simulink model "controller"  (R2019b)
settings: Solver=FixedStepAuto  StartTime=0.0  StopTime=10.0  RelTol=1e-3
undefined symbols (not defined in the file): Kd_mat, Kp_mat
settings Model: Creator=LBRY-SVC-Patron  LastModifiedBy=logan
settings DataIOCC: ReturnWorkspaceOutputs=off
settings OptimizationCC: DefaultParameterBehavior=Inlined  UseDivisionForNetSlopeComputation=on  GainParamInheritBuiltInType=on  UseFloatMulNetSlope=on  InlineInvariantSignals=on  PassReuseOutputArgsAs=Individual arguments  ZeroExternalMemoryAtStartup=off  ZeroInternalMemoryAtStartup=off  NoFixptDivByZeroProtection=on  EfficientFloat2IntCast=on  LifeSpan=1  EfficientTunableParamExpr=on
settings DebuggingCC: ParameterTunabilityLossMsg=error  ArithmeticOperatorsInVariantConditions=warning
settings HardwareCC: ProdLongLongMode=on
settings SFSimCC: SimUseLocalCustomCode=off  MATLABDynamicMemAlloc=off  CustomCodeUndefinedFunction=UseInterfaceOnly
settings RTWCC: SystemTargetFile=ert.tlc  TemplateMakefile=ert_default_tmf  GenerateReport=on  RTWUseLocalCustomCode=off  IncludeHyperlinkInReport=on  LaunchReport=on  TargetLang=C++  GenerateTraceInfo=on  GenerateTraceReport=on  GenerateTraceReportSl=on  GenerateTraceReportSf=on  GenerateTraceReportEml=on
settings CodeAppCC: ForceParamTrailComments=on  IgnoreCustomStorageClasses=off  OperatorAnnotations=on  SimulinkDataObjDesc=on  SFDataObjDesc=on  InsertBlockDesc=on
settings ERTTargetCC: TargetLangStandard=C++03 (ISO)  GenerateSampleERTMain=on  IncludeMdlTerminateFcn=off  CombineSignalStateStructs=on  MultiInstanceERTCode=on  CodeInterfacePackaging=C++ class  SupportComplex=off  SupportContinuousTime=on  InlinedParameterPlacement=NonHierarchical  RootIOFormat=Structure reference  ERTCustomFileTemplate=example_file_process.tlc  ERTFilePackagingFormat=CompactWithDataFile

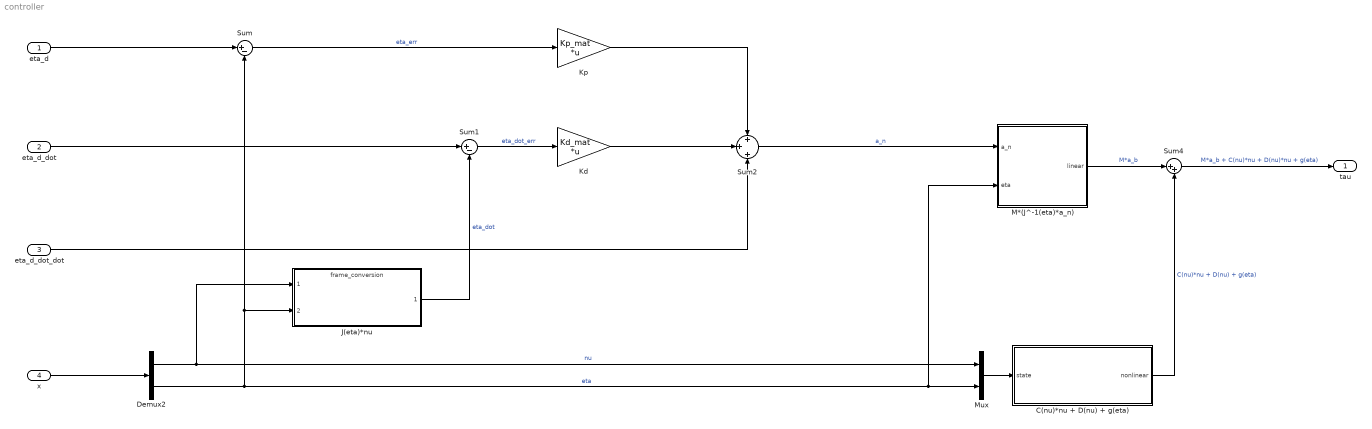
== system controller ==
  eta_d : Inport  PortDimensions=6
  eta_d_dot : Inport  Port=2  PortDimensions=6
  eta_d_dot_dot : Inport  Port=3  PortDimensions=6
  x : Inport  Port=4  PortDimensions=12
  C(nu)*nu + D(nu) + g(eta) : MATLAB Function  TreatAsAtomicUnit=on
  Demux2 : Demux  Outputs=[6,6]
  J(eta)*nu : ModelReference  ModelNameDialog=frame_conversion.slx  SimulationMode=Normal  ModelReferenceVersion=1.22
  "Kd " : Gain  Gain=Kd_mat  Multiplication=Matrix(K*u) (u vector)
  "Kp " : Gain  Gain=Kp_mat  Multiplication=Matrix(K*u) (u vector)  OutDataTypeStr=Inherit: Same as input
  M*(J^-1(eta)*a_n) : MATLAB Function  TreatAsAtomicUnit=on
  Mux : Mux  Inputs=[6,6]
  Sum : Sum  Inputs=|+-
  Sum1 : Sum  Inputs=|+-
  Sum2 : Sum  Inputs=+|+|+
  Sum4 : Sum  Inputs=|++
  "tau " : Outport  PortDimensions=6  VectorParamsAs1DForOutWhenUnconnected=off
  wires:
  x/1 -> Demux2/1
  Demux2/1 -> J(eta)*nu/1, Mux/1  "nu"
  Demux2/2 -> Sum/2, J(eta)*nu/2, M*(J^-1(eta)*a_n)/2(eta), Mux/2  "eta"
  eta_d/1 -> Sum/1
  J(eta)*nu/1 -> Sum1/2  "eta_dot"
  eta_d_dot/1 -> Sum1/1
  Sum1/1 -> "Kd "/1  "eta_dot_err"
  Sum/1 -> "Kp "/1  "eta_err"
  "Kp "/1 -> Sum2/1
  "Kd "/1 -> Sum2/2
  eta_d_dot_dot/1 -> Sum2/3
  Sum2/1 -> M*(J^-1(eta)*a_n)/1(a_n)  "a_n"
  M*(J^-1(eta)*a_n)/1(linear) -> Sum4/1  "M*a_b"
  C(nu)*nu + D(nu) + g(eta)/1(nonlinear) -> Sum4/2  "C(nu)*nu + D(nu) + g(eta)"
  Sum4/1 -> "tau "/1  "M*a_b + C(nu)*nu + D(nu)*nu + g(eta)"
  Mux/1 -> C(nu)*nu + D(nu) + g(eta)/1(state)

== matlab function controller/C(nu)*nu + D(nu) + g(eta) ==
  data: state input; nonlinear output; params parameter
function nonlinear  = feedback_linearization(state, params)
%#codegen

% [nonlinear] = fcn(nu, eta, params) returns the nonlinear terms of the AUV
% model taking rhe previous iterations state

% Load params in to local variables
m = params.m;
W = params.W;
B = params.B; 
Ixx = params.Ixx;
Iyy = params.Iyy;
Izz = params.Izz;
xg = params.xg;
yg = params.yg;
zg = params.zg;
xb = params.xb;
yb = params.yb;
zb = params.zb;
Xu = params.Xu;
Yv = params.Yv;
Zw = params.Zw;
Kp = params.Kp;
Kq = params.Kq;
Nr = params.Nr;
Xuu = params.Xuu;
Yvv = params.Yvv;
Zww = params.Zww;
Kpp = params.Kpp;
Kqq = params.Kqq;
Nrr = params.Nrr;

u = state(1);        % surge velocity          (m/s)
v = state(2);        % sway velocity           (m/s)
w = state(3);        % heave velocity          (m/s)
p = state(4);        % roll velocity           (rad/s)
q = state(5);        % pitch velocity          (rad/s)
r = state(6);        % yaw velocity            (rad/s)
x = state(7);        % position in x-direction (m)
y = state(8);        % position in y-direction (m)
z = state(9);        % position in z-direction (m)
phi = state(10);     % roll angle              (rad)
theta =  state(11);  % pitch angle             (rad)
psi = state(12);     % yaw angle               (rad)

nu  = [u; v; w; p; q; r];          % body frame linear/angluar velocity vector
eta = [x; y; z; phi; theta; psi];  % world frame position/orientation vector

% rigid body coriolis and centripetal matrix 
C_RB = [ 0, 0, 0, 0 m*w, -m*w; ...
         0, 0, 0, -m*w, 0, m*u; ...
         0, 0, 0, m*v, -m*u, 0; ...
         0, m*w, -m*v, 0, Izz*r, -Iyy*q; ...
        -m*w, 0, m*u, -Izz*r, 0, Ixx*p; ...
         m*v, -m*u, 0, Iyy*q, -Ixx*p, 0]; 

% linear drag matrix
D_lin = [ Xu, 0, 0, 0, 0, 0; ...
          0, Yv, 0, 0, 0, 0; ...
          0, 0, Zw, 0, 0, 0; ...
          0, 0, 0, Kp, 0, 0; ...
          0, 0, 0, 0, Kq, 0; ...
          0, 0, 0, 0, 0, Nr ];
      
% quadratic drag matrix
D_quad = [ Xuu*abs(u), 0, 0, 0, 0, 0; ...
           0, Yvv*abs(v), 0, 0, 0, 0; ...
           0, 0, Zww*abs(w), 0, 0, 0; ...
           0, 0, 0, Kpp*abs(p), 0, 0; ...
           0, 0, 0, 0, Kqq*abs(q), 0; ...
           0 ,0 ,0 ,0 ,0, Nrr*abs(r) ];
       
% gravity and bouyancy matrix
g = [ (W-B)*sin(theta); ...
      -(W-B)*cos(theta)*sin(phi); ...
      -(W-B)*cos(theta)*cos(phi); ...
      -(yg*W-yb*B)*cos(theta)*cos(phi) + (zg*W-zb*B)*cos(theta)*sin(phi); ...
      (zg*W-zb*B)*sin(theta) + (xg*W-xb*B)*cos(theta)*cos(phi); ...
      -(xg*W-xb*B)*cos(theta)*sin(phi) - (yg*W-yb*B)*sin(theta) ]; 
 
C = C_RB;
D = D_lin + D_quad;

nonlinear = C*nu + D*nu + g;

end

== matlab function controller/M*(J^-1(eta)*a_n) ==
  data: a_n input; eta input; linear output; params parameter
function linear  = J_inv_times_M(a_n, eta, params)
%#codegen

% [linear] = J_inv_times_M(eta, params) returns the linear result
% of the controller, namely M*a_b where a_b = J^-1(eta)*a_n and a_b, a_n
% are the commanded accelerations in body and world frame respectively.

% Load params in to local variables
m = params.m;
Ixx = params.Ixx;
Iyy = params.Iyy;
Izz = params.Izz;

x = eta(1);        % position in x-direction (m)
y = eta(2);        % position in y-direction (m)
z = eta(3);        % position in z-direction (m)
phi = eta(4);      % roll angle              (rad)
theta =  eta(5);   % pitch angle             (rad)
psi = eta(6);      % yaw angle               (rad)

% rigid body mass and inertia matrix
M_RB = [ m, 0, 0, 0, 0, 0; ...
         0, m, 0, 0, 0, 0; ...
         0, 0, m, 0, 0, 0; ...
         0, 0, 0, Ixx, 0, 0; ...
         0, 0, 0, 0, Iyy, 0; ...
         0, 0, 0, 0, 0, Izz ]; 
  
M = M_RB;

% Calculate rotation matrix J used to convert nu to world frame
cphi = cos(phi);
sphi = sin(phi);
cth  = cos(theta);
sth  = sin(theta);
cpsi = cos(psi);
spsi = sin(psi);

J1 = [...
   cpsi*cth  -spsi*cphi+cpsi*sth*sphi  spsi*sphi+cpsi*cphi*sth
   spsi*cth  cpsi*cphi+sphi*sth*spsi   -cpsi*sphi+sth*spsi*cphi
   -sth      cth*sphi                  cth*cphi ];

if cth==0, error('J2 is singular for theta = +-90 degrees'); end
 
J2 = [...
      1  sphi*sth/cth  cphi*sth/cth;
      0  cphi          -sphi;
      0  sphi/cth      cphi/cth ];
  
J = [ J1  zeros(3,3);
      zeros(3,3) J2 ];

% Note that transpose(J) = inv(J)
linear = M*transpose(J)*a_n;

end
